simulink model "cm_ldpc_decode_qpsk"  (R2022a)
settings: Solver=VariableStepAuto  StartTime=0.0  StopTime=0  RelTol=1e-3
InitFcn:
  | snr = 1.0;
undefined symbols (not defined in the file or in its folder): dvbs2ldpc
libraries: commblkcod2 x2, commdigbbndpm3 x2, commchan3 x1, commsink2 x1
settings Model: Creator=The MathWorks, Inc.  LastModifiedBy=user
settings SolverCC: AlgebraicLoopSolver=TrustRegion
settings DataIOCC: ReturnWorkspaceOutputs=off
settings DebuggingCC: UnconnectedInputMsg=warning  UnconnectedOutputMsg=warning  UnconnectedLineMsg=warning  SFMachineParentedDataDiag=warning  ArithmeticOperatorsInVariantConditions=warning
settings SFSimCC: SimUseLocalCustomCode=off  CustomCodeUndefinedFunction=UseInterfaceOnly
settings RTWCC: RTWUseLocalCustomCode=off
settings CodeAppCC: StateflowObjectComments=on
settings GRTTargetCC: TargetLangStandard=C89/C90 (ANSI)
settings ConfigComp: CovMetricSettings=dsw  CovSaveCumulativeToWorkspaceVar=on  CovSaveSingleToWorkspaceVar=on  CovExternalEMLEnable=off

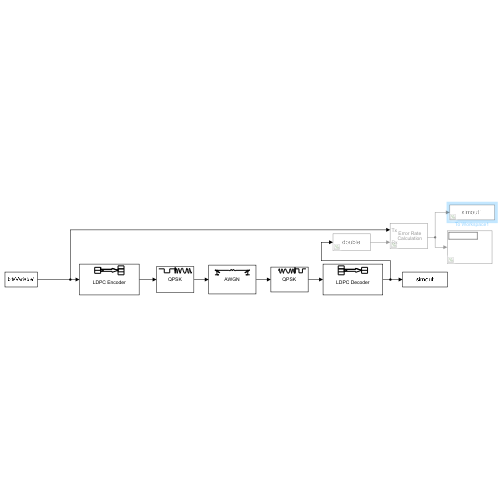
[thumbnail: Simulink's stored preview of the top-level diagram]
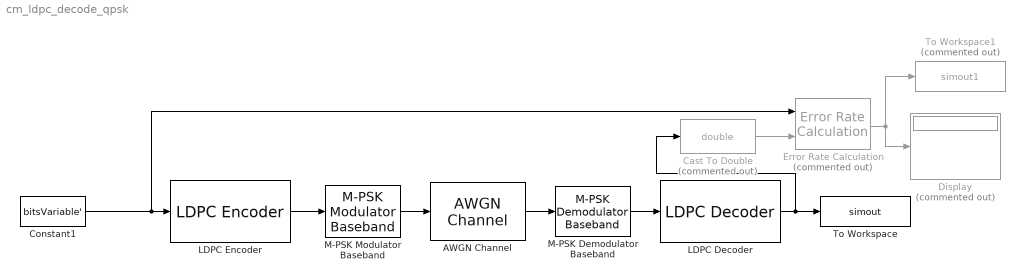
== system cm_ldpc_decode_qpsk ==
  AWGN Channel : commchan3/AWGN Channel  InputProcessing=Columns as channels (frame based)  seed=randi([0 1000])  noiseMode="Signal to noise ratio  (Eb/No)"  EbNodB=ebno  EsNodB=10  SNRdB=ebno  bitsPerSym=2  Ps=1  Tsym=2  variance=1
  Cast To Double : DataTypeConversion  Commented=on  OutDataTypeStr=double  SaturateOnIntegerOverflow=off  RndMeth=Floor
  Constant1 : Constant  Value=bitsVariable'  SampleTime=1
  Display : Display  Commented=on
  Error Rate Calculation : commsink2/Error Rate Calculation  Commented=on  N=0  st_delay=0  cp_mode=Entire frame  subframe=[]  PMode=Port  WsName=BERQPSK  RsMode2=off  stop=off  numErr=100  maxBits=1e6
  LDPC Decoder : commblkcod2/LDPC Decoder  ParityCheckMat=dvbs2ldpc(9/10)  OutputFmt=Information part  DecisionType=Hard decision  OutputDataType=boolean  NumIter=50  DoParityCheck=off  OutputNumIter=off  OutputFinalChecks=off
      settings: SourceProductBaseCode=CM
  LDPC Encoder : commblkcod2/LDPC Encoder  ParityCheckMat=dvbs2ldpc(9/10)
      settings: SourceProductBaseCode=CM
  M-PSK Demodulator Baseband : commdigbbndpm3/M-PSK Demodulator Baseband  M=4  OutType=Bit  DecType=Approximate log-likelihood ratio  VarSource=Dialog  Variance=1  Dec=Gray  Mapping=[0:7]  Ph=pi/4  outDtype1=Inherit via internal rule  outDtype2=Inherit via internal rule  derotateFactorWordLen=16  derotateFactorDataTypeStr=Inherit: Same word length as input  derotateFactorLastDataTypeStr=Inherit: Same word length as input
  M-PSK Modulator Baseband : commdigbbndpm3/M-PSK Modulator Baseband  M=4  InType=Bit  Enc=Gray  Mapping=[0:7]  Ph=pi/4  outDtype=double  outWordLen=16  outUDDataType=sfix(16)  outFracLenMode=Best precision  outFracLen=15  outDataTypeStr=double  outLastDataTypeStr=double
  To Workspace : ToWorkspace  VariableName=simout  SampleTime=-1
      settings: Save2DSignal=2-D array (concatenate along first dimension)
  To Workspace1 : ToWorkspace  Commented=on  VariableName=simout1  SampleTime=-1
  wires:
  LDPC Decoder/1 -> Cast To Double/1, To Workspace/1
  Constant1/1 -> Error Rate Calculation/1, LDPC Encoder/1
  M-PSK Modulator Baseband/1 -> AWGN Channel/1
  LDPC Encoder/1 -> M-PSK Modulator Baseband/1
  M-PSK Demodulator Baseband/1 -> LDPC Decoder/1
  AWGN Channel/1 -> M-PSK Demodulator Baseband/1
  Cast To Double/1 -> Error Rate Calculation/2
  Error Rate Calculation/1 -> To Workspace1/1, Display/1
